simulink model "FD"  (R2019b)
settings: Solver=VariableStepAuto  StartTime=0.0  StopTime=10  RelTol=1e-3
values from neighbouring files (symbols this model uses):
  A = -2    [computation.m]
  A_F = A+L*C    [computation.m]
  B = 1    [computation.m]
  Bd = [4,-4]    [computation.m]
  Bf = 1    [computation.m]
  C = [4;-5]    [computation.m]
  C_F = H*C    [computation.m]
  D = [0;0]    [computation.m]
  Dd = [-4,0;3,2]    [computation.m]
  Df = [6;1]    [computation.m]
  H = Df1+S*Df2    [computation.m]
  L = L-X*(H*C)'*H    [computation.m]
libraries: simulink x1
settings Model: Creator=cz  LastModifiedBy=cz

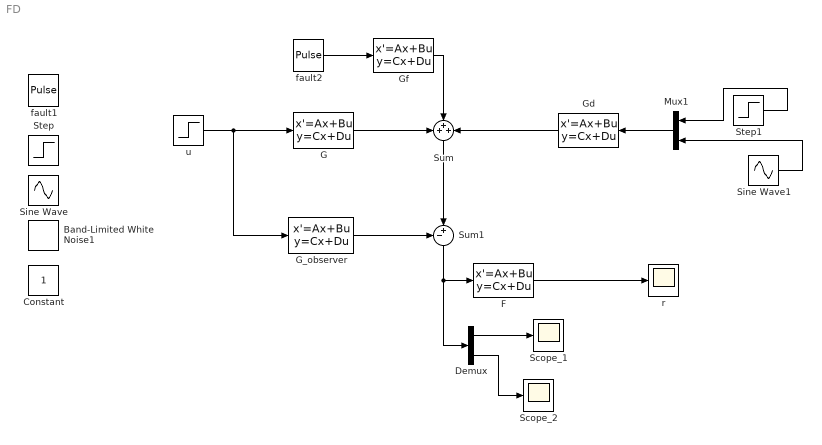
== system FD ==
  Band-Limited White Noise1 : simulink/Sources/Band-Limited White Noise  Cov=[0.1]  Ts=0.1  seed=[23341]
  Constant : Constant
  Demux : Demux  Outputs=2
  F : StateSpace  A=A_F  B=L  C=C_F  D=H  InitialCondition=0
  G : StateSpace  A=A  B=B  C=C  D=D  InitialCondition=0
  G_observer : StateSpace  A=A  B=B  C=C  D=D  InitialCondition=0
  Gd : StateSpace  A=A  B=Bd  C=C  D=Dd  InitialCondition=0
  Gf : StateSpace  A=A  B=Bf  C=C  D=Df  InitialCondition=0
  Mux1 : Mux  Inputs=2
  Scope_1 : Scope
  Scope_2 : Scope
  Sine Wave : Sin  SampleTime=0
  Sine Wave1 : Sin  SampleTime=0
  Step : Step  SampleTime=0
  Step1 : Step  Time=2  SampleTime=0
  Sum : Sum  Inputs=+++
  Sum1 : Sum  Inputs=-+|
  fault1 : DiscretePulseGenerator  PulseType=Time based  Period=1  PulseWidth=50  PhaseDelay=6
  fault2 : DiscretePulseGenerator  PulseType=Time based  Period=1  PulseWidth=50  PhaseDelay=6
  r : Scope
  u : Step  SampleTime=0
  wires:
  u/1 -> G_observer/1, G/1
  G/1 -> Sum/1
  Gf/1 -> Sum/2
  Gd/1 -> Sum/3
  Mux1/1 -> Gd/1
  Sum/1 -> Sum1/2
  G_observer/1 -> Sum1/1
  Demux/1 -> Scope_1/1
  Demux/2 -> Scope_2/1
  Step1/1 -> Mux1/1
  fault2/1 -> Gf/1
  Sine Wave1/1 -> Mux1/2
  Sum1/1 -> Demux/1, F/1
  F/1 -> r/1
